simulink model "Tipologia3_simulink"  (R2014a)
settings: Solver=ode45  StartTime=0.0  StopTime=10.0  RelTol=1e-3
values from neighbouring files (symbols this model uses):
  A = 9    [Tipologia3.m]
  d2 = 4    [Tipologia1.m]    (also in Tipologia1_v2.m; Tipologia3.m = 0.0055)
libraries: cstblocks x2, simulink x2
settings Model: Creator=giova  LastModifiedBy=giova

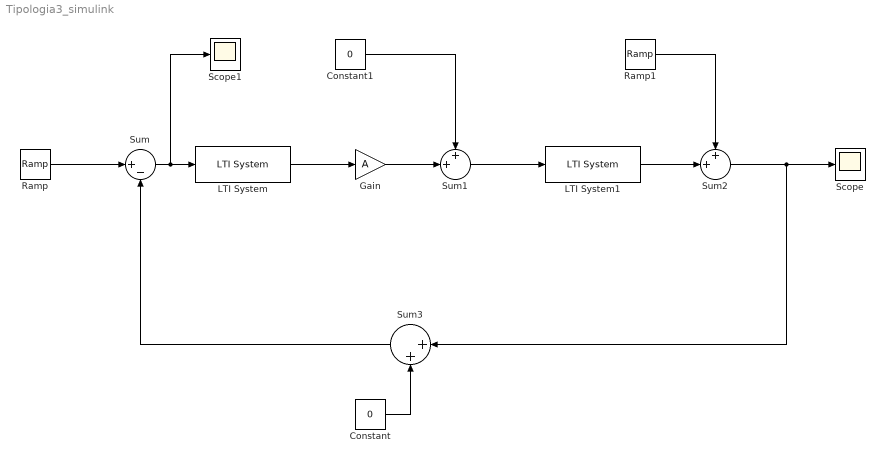
== system Tipologia3_simulink ==
  Constant : Constant  Value=0
  Constant1 : Constant  Value=0
  Gain : Gain  Gain=A
  LTI System : cstblocks/LTI System  sys=C  IC=[]
  LTI System1 : cstblocks/LTI System  sys=F  IC=[]
  Ramp : simulink/Sources/Ramp  slope=0  start=0  X0=0
  Ramp1 : simulink/Sources/Ramp  slope=d2  start=0  X0=0
  Scope : Scope
  Scope1 : Scope
  Sum : Sum  Inputs=|+-
  Sum1 : Sum  Inputs=++|
  Sum2 : Sum  Inputs=++|
  Sum3 : Sum  Inputs=|++
  wires:
  Sum/1 -> Scope1/1, LTI System/1
  LTI System/1 -> Gain/1
  Gain/1 -> Sum1/2
  Sum1/1 -> LTI System1/1
  LTI System1/1 -> Sum2/2
  Sum2/1 -> Sum3/1, Scope/1
  Sum3/1 -> Sum/2
  Constant/1 -> Sum3/2
  Ramp1/1 -> Sum2/1
  Constant1/1 -> Sum1/1
  Ramp/1 -> Sum/1
